simulink model "Channel_Picking_6_of_20"  (R2023a)
settings: Solver=ode23tb  StartTime=0.0  StopTime=3.0  RelTol=1e-3
libraries: dspfdesign x21, dspindex x4, dspvision x2, dspstat3 x1
settings Model: Creator=zacha  LastModifiedBy=zacha
settings DebuggingCC: UnconnectedInputMsg=warning  UnconnectedOutputMsg=warning  UnconnectedLineMsg=warning
settings ModelReferenceCC: EnableRefExpFcnMdlSchedulingChecks=on
settings RTWCC: DLArmComputeVersion=19.05

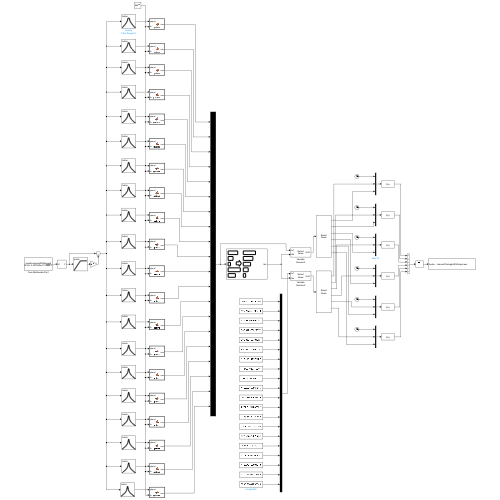
[thumbnail: Simulink's stored preview of the top-level diagram]
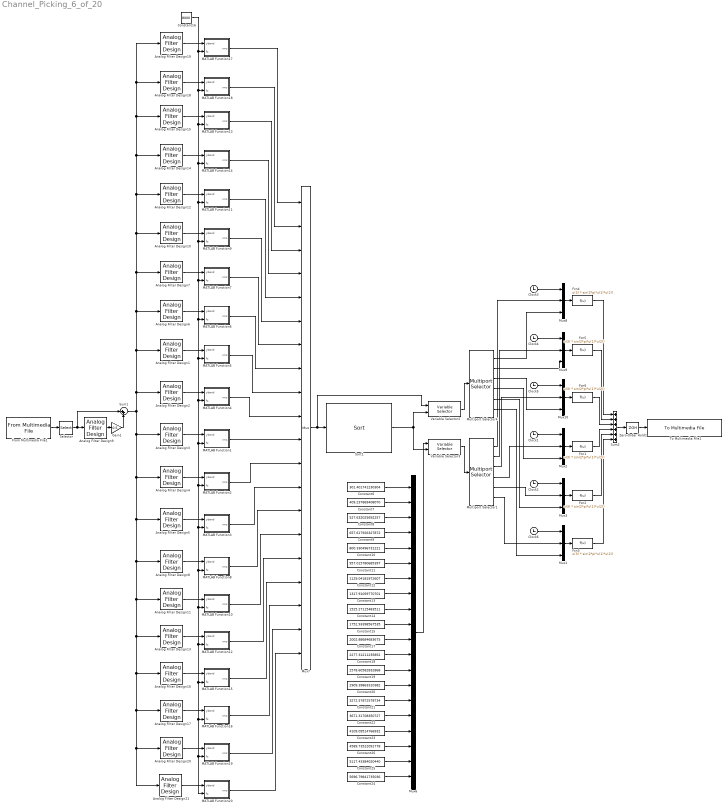
== system Channel_Picking_6_of_20 ==
  Analog Filter Design1 : dspfdesign/Analog Filter Design  method=Butterworth  filttype=Bandpass  N=6  Wlo=8901.71649069657  Whi=10265.4061283531  Rp=2  Rs=40
  Analog Filter Design10 : dspfdesign/Analog Filter Design  method=Butterworth  filttype=Bandpass  N=6  Wlo=5497.89355477605  Whi=6528.32142910693  Rp=2  Rs=40
  Analog Filter Design11 : dspfdesign/Analog Filter Design  method=Butterworth  filttype=Bandpass  N=6  Wlo=19368.0065720074  Whi=21756.4305609036  Rp=2  Rs=40
  Analog Filter Design12 : dspfdesign/Analog Filter Design  method=Butterworth  filttype=Bandpass  N=6  Wlo=4559.35608112265  Whi=5497.89355477605  Rp=2  Rs=40
  Analog Filter Design13 : dspfdesign/Analog Filter Design  method=Butterworth  filttype=Bandpass  N=6  Wlo=21756.4305609036  Whi=24378.7005532769  Rp=2  Rs=40
  Analog Filter Design14 : dspfdesign/Analog Filter Design  method=Butterworth  filttype=Bandpass  N=6  Wlo=3704.51450375974  Whi=4559.35608112265  Rp=2  Rs=40
  Analog Filter Design15 : dspfdesign/Analog Filter Design  method=Butterworth  filttype=Bandpass  N=6  Wlo=2925.90507909423  Whi=3704.51450375974  Rp=2  Rs=40
  Analog Filter Design16 : dspfdesign/Analog Filter Design  method=Butterworth  filttype=Bandpass  N=6  Wlo=24378.7005532769  Whi=27257.7119620007  Rp=2  Rs=40
  Analog Filter Design17 : dspfdesign/Analog Filter Design  method=Butterworth  filttype=Bandpass  N=6  Wlo=27257.7119620007  Whi=30418.6018458298  Rp=2  Rs=40
  Analog Filter Design18 : dspfdesign/Analog Filter Design  method=Butterworth  filttype=Bandpass  N=6  Wlo=2216.72965731829  Whi=2925.90507909423  Rp=2  Rs=40
  Analog Filter Design19 : dspfdesign/Analog Filter Design  method=Butterworth  filttype=Bandpass  N=6  Wlo=1570.79632679490  Whi=2216.72965731829  Rp=2  Rs=40
  Analog Filter Design2 : dspfdesign/Analog Filter Design  method=Butterworth  filttype=Bandpass  N=6  Wlo=10265.4061283531  Whi=11762.6119981492  Rp=2  Rs=40
  Analog Filter Design20 : dspfdesign/Analog Filter Design  method=Butterworth  filttype=Bandpass  N=6  Wlo=30418.6018458298  Whi=33888.9683846419  Rp=2  Rs=40
  Analog Filter Design21 : dspfdesign/Analog Filter Design  method=Butterworth  filttype=Bandpass  N=6  Wlo=33888.9683846419  Whi=37699.1118430775  Rp=2  Rs=40
  Analog Filter Design3 : dspfdesign/Analog Filter Design  method=Butterworth  filttype=Bandpass  N=6  Wlo=11762.6119981492  Whi=13406.4064178267  Rp=2  Rs=40
  Analog Filter Design4 : dspfdesign/Analog Filter Design  method=Butterworth  filttype=Bandpass  N=6  Wlo=13406.4064178267  Whi=15211.1415906396  Rp=2  Rs=40
  Analog Filter Design5 : dspfdesign/Analog Filter Design  method=Butterworth  filttype=Bandpass  N=6  Wlo=15211.1415906396  Whi=17192.5749164852  Rp=2  Rs=40
  Analog Filter Design6 : dspfdesign/Analog Filter Design  method=Butterworth  filttype=Bandpass  N=6  Wlo=7659.63651668133  Whi=8901.71649069657  Rp=2  Rs=40
  Analog Filter Design7 : dspfdesign/Analog Filter Design  method=Butterworth  filttype=Bandpass  N=6  Wlo=6528.32142910693  Whi=7659.63651668133  Rp=2  Rs=40
  Analog Filter Design8 : dspfdesign/Analog Filter Design  method=Butterworth  filttype=Bandpass  N=6  Wlo=17192.5749164852  Whi=19368.0065720074  Rp=2  Rs=40
  Analog Filter Design9 : dspfdesign/Analog Filter Design  method=Butterworth  filttype=Highpass  N=6  Wlo=7539.82236  Whi=80  Rp=2  Rs=40
  Clock{1..6} (6 alike) : Clock
  Constant10 : Constant  Value=800.330496731221
  Constant11 : Constant  Value=957.015780685397
  Constant12 : Constant  Value=1129.04181972607
  Constant13 : Constant  Value=1317.91059770701
  Constant14 : Constant  Value=1525.27115483511
  Constant15 : Constant  Value=1752.93398567535
  Constant16 : Constant  Value=8000
  Constant17 : Constant  Value=2002.88684683675
  Constant18 : Constant  Value=2277.31211235852
  Constant19 : Constant  Value=2578.60582832868
  Constant20 : Constant  Value=2909.39863310382
  Constant21 : Constant  Value=3272.57872578734
  Constant22 : Constant  Value=3671.31708350727
  Constant23 : Constant  Value=4109.09514766932
  Constant24 : Constant  Value=5696.79841735036
  Constant25 : Constant  Value=5117.43384020440
  Constant26 : Constant  Value=4589.73522091778
  Constant6 : Constant  Value=301.401741230304
  Constant7 : Constant  Value=409.237869408070
  Constant8 : Constant  Value=527.632025692257
  Constant9 : Constant  Value=657.617926327872
  Fcn{1..6} (6 alike) : Fcn  Expr=u(3) * sin(2*pi*u(1)*u(2))
  From Multimedia File1 : dspvision/From Multimedia File  inputFilename=C:\Users\zacha\Desktop\Cochlear\Media\inputSentance8000hz.mp3  readRange=[1 Inf]  loop=on  numPlays=1  outputStreams=Audio only  videoDataType=single  audioDataType=double  inheritSampleTime=off  userDefinedSampleTime=1/8000  noAudioOutput=off  isIntensityVideo=off  fourcc=RGB  colorVideoFormat=Separate color signals  outputEOF=off  dataOrg=Column-major  audioFrameSize=1  computeAudioFrameSize=off  outSamplingMode=Sample based
      settings: LibrarySourceBlock=dspsrcs4/From Multimedia File
  Gain1 : Gain  Gain=0.5
  MATLAB Function1 : MATLAB Function  TreatAsAtomicUnit=on
  MATLAB Function10 : MATLAB Function  TreatAsAtomicUnit=on
  MATLAB Function11 : MATLAB Function  TreatAsAtomicUnit=on
  MATLAB Function12 : MATLAB Function  TreatAsAtomicUnit=on
  MATLAB Function13 : MATLAB Function  TreatAsAtomicUnit=on
  MATLAB Function14 : MATLAB Function  TreatAsAtomicUnit=on
  MATLAB Function15 : MATLAB Function  TreatAsAtomicUnit=on
  MATLAB Function16 : MATLAB Function  TreatAsAtomicUnit=on
  MATLAB Function17 : MATLAB Function  TreatAsAtomicUnit=on
  MATLAB Function18 : MATLAB Function  TreatAsAtomicUnit=on
  MATLAB Function19 : MATLAB Function  TreatAsAtomicUnit=on
  MATLAB Function2 : MATLAB Function  TreatAsAtomicUnit=on
  MATLAB Function20 : MATLAB Function  TreatAsAtomicUnit=on
  MATLAB Function3 : MATLAB Function  TreatAsAtomicUnit=on
  MATLAB Function4 : MATLAB Function  TreatAsAtomicUnit=on
  MATLAB Function5 : MATLAB Function  TreatAsAtomicUnit=on
  MATLAB Function6 : MATLAB Function  TreatAsAtomicUnit=on
  MATLAB Function7 : MATLAB Function  TreatAsAtomicUnit=on
  MATLAB Function8 : MATLAB Function  TreatAsAtomicUnit=on
  MATLAB Function9 : MATLAB Function  TreatAsAtomicUnit=on
  Multiport Selector1 : dspindex/Multiport Selector  rowsOrCols=Rows  idxCellArray={ 1, 2,3,4,5,6 }  idxErrMode=Clip Index
  Multiport Selector4 : dspindex/Multiport Selector  rowsOrCols=Rows  idxCellArray={ 1, 2,3,4,5,6 }  idxErrMode=Clip Index
  Mux{1..3,8..10} (6 alike) : Mux  Inputs=3
  Mux6 : Mux  Inputs=20
  Mux7 : Mux  Inputs=20
  Selector : Selector  NumberOfDimensions=2  InputPortWidth=3  IndexOptions=Select all,Index vector (dialog)  Indices=[2],1  OutputSizes=1,1
  Sort1 : dspstat3/Sort  otype=Index  dir=Descending  sortAlg=Quick sort  roundingMode=Floor  overflowMode=off  accumDataTypeStr=Inherit: Same as product output  accumLastDataTypeStr=Inherit: Same as product output
  Sum1 : Sum  Inputs=|++
  Sum2 : Sum  Inputs=++++++
  To Multimedia File1 : dspvision/To Multimedia File  outputFilename=C:\Users\zacha\Desktop\Cochlear\Media\channelPicking6of20Output.wav  streamSelection=Audio only  videoCompressor=None (uncompressed)  audioCompressor=None (uncompressed)  imagePorts=Separate color signals  fileType=WAV  audioDatatype=16-bit integer  fourcc=RGB  videoQuality=75  mj2000CompFactor=10
      settings: LibrarySourceBlock=dspsnks4/To Multimedia File
  Variable Selector2 : dspindex/Variable Selector  NumInputs=1  rowsOrCols=Rows  IdxMode=Variable  Elements=[1 3]  ZerOneIdxMode=One-based  errmode=Clip Index  FillMode=on  FillValues=0
      settings: LibrarySourceBlock=|
      | dsphdlsupportsigmgmt/Variable
      | Selector
  Variable Selector3 : dspindex/Variable Selector  NumInputs=1  rowsOrCols=Rows  IdxMode=Variable  Elements=[1 3]  ZerOneIdxMode=One-based  errmode=Clip Index  FillMode=on  FillValues=0
      settings: LibrarySourceBlock=|
      | dsphdlsupportsigmgmt/Variable
      | Selector
  Zero-Order Hold1 : ZeroOrderHold  SampleTime=1/8000
  wires:
  Analog Filter Design20/1 -> MATLAB Function19/1(yband)
  Analog Filter Design21/1 -> MATLAB Function20/1(yband)
  Sum1/1 -> Analog Filter Design19/1, Analog Filter Design18/1, Analog Filter Design15/1, Analog Filter Design14/1, Analog Filter Design12/1, Analog Filter Design10/1, Analog Filter Design7/1, Analog Filter Design6/1, Analog Filter Design1/1, Analog Filter Design2/1, Analog Filter Design21/1, Analog Filter Design20/1, Analog Filter Design17/1, Analog Filter Design16/1, Analog Filter Design13/1, Analog Filter Design11/1, Analog Filter Design8/1, Analog Filter Design5/1, Analog Filter Design4/1, Analog Filter Design3/1
  Analog Filter Design8/1 -> MATLAB Function8/1(yband)
  Analog Filter Design10/1 -> MATLAB Function9/1(yband)
  Analog Filter Design6/1 -> MATLAB Function6/1(yband)
  Analog Filter Design3/1 -> MATLAB Function1/1(yband)
  Analog Filter Design13/1 -> MATLAB Function12/1(yband)
  Analog Filter Design2/1 -> MATLAB Function4/1(yband)
  Analog Filter Design15/1 -> MATLAB Function13/1(yband)
  Analog Filter Design12/1 -> MATLAB Function11/1(yband)
  Analog Filter Design4/1 -> MATLAB Function2/1(yband)
  Analog Filter Design7/1 -> MATLAB Function7/1(yband)
  Analog Filter Design11/1 -> MATLAB Function10/1(yband)
  Analog Filter Design9/1 -> Gain1/1
  Analog Filter Design19/1 -> MATLAB Function17/1(yband)
  Analog Filter Design5/1 -> MATLAB Function3/1(yband)
  Constant16/1 -> MATLAB Function20/2(fs), MATLAB Function19/2(fs), MATLAB Function16/2(fs), MATLAB Function15/2(fs), MATLAB Function12/2(fs), MATLAB Function10/2(fs), MATLAB Function8/2(fs), MATLAB Function3/2(fs), MATLAB Function2/2(fs), MATLAB Function1/2(fs), MATLAB Function4/2(fs), MATLAB Function5/2(fs), MATLAB Function6/2(fs), MATLAB Function7/2(fs), MATLAB Function9/2(fs), MATLAB Function11/2(fs), MATLAB Function14/2(fs), MATLAB Function13/2(fs), MATLAB Function18/2(fs), MATLAB Function17/2(fs)
  Analog Filter Design18/1 -> MATLAB Function18/1(yband)
  Analog Filter Design1/1 -> MATLAB Function5/1(yband)
  Analog Filter Design16/1 -> MATLAB Function15/1(yband)
  Analog Filter Design14/1 -> MATLAB Function14/1(yband)
  Analog Filter Design17/1 -> MATLAB Function16/1(yband)
  From Multimedia File1/1 -> Selector/1
  Gain1/1 -> Sum1/2
  Selector/1 -> Analog Filter Design9/1, Sum1/1
  Constant6/1 -> Mux6/1
  Constant7/1 -> Mux6/2
  Constant8/1 -> Mux6/3
  Constant9/1 -> Mux6/4
  Constant10/1 -> Mux6/5
  Constant11/1 -> Mux6/6
  Constant12/1 -> Mux6/7
  Constant13/1 -> Mux6/8
  Constant14/1 -> Mux6/9
  Constant15/1 -> Mux6/10
  Constant17/1 -> Mux6/11
  Constant18/1 -> Mux6/12
  Constant19/1 -> Mux6/13
  Constant20/1 -> Mux6/14
  Constant21/1 -> Mux6/15
  Constant22/1 -> Mux6/16
  Constant23/1 -> Mux6/17
  Constant26/1 -> Mux6/18
  Constant25/1 -> Mux6/19
  Constant24/1 -> Mux6/20
  MATLAB Function17/1(rms) -> Mux7/1
  MATLAB Function18/1(rms) -> Mux7/2
  MATLAB Function13/1(rms) -> Mux7/3
  MATLAB Function14/1(rms) -> Mux7/4
  MATLAB Function11/1(rms) -> Mux7/5
  MATLAB Function9/1(rms) -> Mux7/6
  MATLAB Function7/1(rms) -> Mux7/7
  MATLAB Function6/1(rms) -> Mux7/8
  MATLAB Function5/1(rms) -> Mux7/9
  MATLAB Function4/1(rms) -> Mux7/10
  MATLAB Function1/1(rms) -> Mux7/11
  MATLAB Function2/1(rms) -> Mux7/12
  MATLAB Function3/1(rms) -> Mux7/13
  MATLAB Function8/1(rms) -> Mux7/14
  MATLAB Function10/1(rms) -> Mux7/15
  MATLAB Function12/1(rms) -> Mux7/16
  MATLAB Function15/1(rms) -> Mux7/17
  MATLAB Function16/1(rms) -> Mux7/18
  MATLAB Function19/1(rms) -> Mux7/19
  MATLAB Function20/1(rms) -> Mux7/20
  Mux7/1 -> Variable Selector2/1, Sort1/1
  Variable Selector2/1 -> Multiport Selector4/1
  Variable Selector3/1 -> Multiport Selector1/1
  Sort1/1 -> Variable Selector2/2, Variable Selector3/2
  Mux6/1 -> Variable Selector3/1
  Mux9/1 -> Fcn5/1
  Clock4/1 -> Mux9/1
  Fcn4/1 -> Sum2/1
  Sum2/1 -> Zero-Order Hold1/1
  Clock3/1 -> Mux8/1
  Mux8/1 -> Fcn4/1
  Fcn6/1 -> Sum2/3
  Fcn5/1 -> Sum2/2
  Zero-Order Hold1/1 -> To Multimedia File1/1
  Clock5/1 -> Mux10/1
  Mux10/1 -> Fcn6/1
  Clock6/1 -> Mux1/1
  Mux3/1 -> Fcn2/1
  Mux2/1 -> Fcn1/1
  Clock2/1 -> Mux3/1
  Clock1/1 -> Mux2/1
  Mux1/1 -> Fcn3/1
  Fcn1/1 -> Sum2/4
  Fcn2/1 -> Sum2/5
  Fcn3/1 -> Sum2/6
  Multiport Selector4/1 -> Mux8/3
  Multiport Selector4/2 -> Mux9/3
  Multiport Selector4/3 -> Mux10/3
  Multiport Selector4/4 -> Mux2/3
  Multiport Selector4/5 -> Mux3/3
  Multiport Selector4/6 -> Mux1/3
  Multiport Selector1/1 -> Mux8/2
  Multiport Selector1/2 -> Mux9/2
  Multiport Selector1/3 -> Mux10/2
  Multiport Selector1/4 -> Mux2/2
  Multiport Selector1/5 -> Mux3/2
  Multiport Selector1/6 -> Mux1/2

== matlab function Channel_Picking_6_of_20/MATLAB Function13 ==
  data: yband input; rms output; fs input
function rms = getrms(yband,fs)

    y = abs(yband); %rectifying it makes it sound bad

    [b,a] = butter(2,400/(fs/2));

    z = filter(b,a,y); %this filter also makes it sound bad

    windowsize = round(4/(1000/fs)); %rms computed every 4ms = windowsize samples

    [yupper,ylower] = envelope(yband,windowsize,'rms'); %changed to yband here

    %envelope(z,windowsize,'rms');

    rms = yupper;
end

== matlab function Channel_Picking_6_of_20/MATLAB Function14 ==
  data: yband input; rms output; fs input
function rms = getrms(yband,fs)

    y = abs(yband); %rectifying it makes it sound bad

    [b,a] = butter(2,400/(fs/2));

    z = filter(b,a,y); %this filter also makes it sound bad

    windowsize = round(4/(1000/fs)); %rms computed every 4ms = windowsize samples

    [yupper,ylower] = envelope(yband,windowsize,'rms'); %changed to yband here

    %envelope(z,windowsize,'rms');

    rms = yupper;
end

== matlab function Channel_Picking_6_of_20/MATLAB Function15 ==
  data: yband input; rms output; fs input
function rms = getrms(yband,fs)

    y = abs(yband); %rectifying it makes it sound bad

    [b,a] = butter(2,400/(fs/2));

    z = filter(b,a,y); %this filter also makes it sound bad

    windowsize = round(4/(1000/fs)); %rms computed every 4ms = windowsize samples

    [yupper,ylower] = envelope(yband,windowsize,'rms'); %changed to yband here

    %envelope(z,windowsize,'rms');

    rms = yupper;
end

== matlab function Channel_Picking_6_of_20/MATLAB Function16 ==
  data: yband input; rms output; fs input
function rms = getrms(yband,fs)

    y = abs(yband); %rectifying it makes it sound bad

    [b,a] = butter(2,400/(fs/2));

    z = filter(b,a,y); %this filter also makes it sound bad

    windowsize = round(4/(1000/fs)); %rms computed every 4ms = windowsize samples

    [yupper,ylower] = envelope(yband,windowsize,'rms'); %changed to yband here

    %envelope(z,windowsize,'rms');

    rms = yupper;
end

== matlab function Channel_Picking_6_of_20/MATLAB Function17 ==
  data: yband input; rms output; fs input
function rms = getrms(yband,fs)

    y = abs(yband); %rectifying it makes it sound bad

    [b,a] = butter(2,400/(fs/2));

    z = filter(b,a,y); %this filter also makes it sound bad

    windowsize = round(4/(1000/fs)); %rms computed every 4ms = windowsize samples

    [yupper,ylower] = envelope(yband,windowsize,'rms'); %changed to yband here

    %envelope(z,windowsize,'rms');

    rms = yupper;
end

== matlab function Channel_Picking_6_of_20/MATLAB Function18 ==
  data: yband input; rms output; fs input
function rms = getrms(yband,fs)

    y = abs(yband); %rectifying it makes it sound bad

    [b,a] = butter(2,400/(fs/2));

    z = filter(b,a,y); %this filter also makes it sound bad

    windowsize = round(4/(1000/fs)); %rms computed every 4ms = windowsize samples

    [yupper,ylower] = envelope(yband,windowsize,'rms'); %changed to yband here

    %envelope(z,windowsize,'rms');

    rms = yupper;
end

== matlab function Channel_Picking_6_of_20/MATLAB Function19 ==
  data: yband input; rms output; fs input
function rms = getrms(yband,fs)

    y = abs(yband); %rectifying it makes it sound bad

    [b,a] = butter(2,400/(fs/2));

    z = filter(b,a,y); %this filter also makes it sound bad

    windowsize = round(4/(1000/fs)); %rms computed every 4ms = windowsize samples

    [yupper,ylower] = envelope(yband,windowsize,'rms'); %changed to yband here

    %envelope(z,windowsize,'rms');

    rms = yupper;
end

== matlab function Channel_Picking_6_of_20/MATLAB Function20 ==
  data: yband input; rms output; fs input
function rms = getrms(yband,fs)

    y = abs(yband); %rectifying it makes it sound bad

    [b,a] = butter(2,400/(fs/2));

    z = filter(b,a,y); %this filter also makes it sound bad

    windowsize = round(4/(1000/fs)); %rms computed every 4ms = windowsize samples

    [yupper,ylower] = envelope(yband,windowsize,'rms'); %changed to yband here

    %envelope(z,windowsize,'rms');

    rms = yupper;
end

== matlab function Channel_Picking_6_of_20/MATLAB Function2 ==
  data: yband input; rms output; fs input
function rms = getrms(yband,fs)

    y = abs(yband); %rectifying it makes it sound bad

    [b,a] = butter(2,400/(fs/2));

    z = filter(b,a,y); %this filter also makes it sound bad

    windowsize = round(4/(1000/fs)); %rms computed every 4ms = windowsize samples

    [yupper,ylower] = envelope(yband,windowsize,'rms'); %changed to yband here

    %envelope(z,windowsize,'rms');

    rms = yupper;
end

== matlab function Channel_Picking_6_of_20/MATLAB Function3 ==
  data: yband input; rms output; fs input
function rms = getrms(yband,fs)

    y = abs(yband); %rectifying it makes it sound bad

    [b,a] = butter(2,400/(fs/2));

    z = filter(b,a,y); %this filter also makes it sound bad

    windowsize = round(4/(1000/fs)); %rms computed every 4ms = windowsize samples

    [yupper,ylower] = envelope(yband,windowsize,'rms'); %changed to yband here

    %envelope(z,windowsize,'rms');

    rms = yupper;
end

== matlab function Channel_Picking_6_of_20/MATLAB Function6 ==
  data: yband input; rms output; fs input
function rms = getrms(yband,fs)

    y = abs(yband); %rectifying it makes it sound bad

    [b,a] = butter(2,400/(fs/2));

    z = filter(b,a,y); %this filter also makes it sound bad

    windowsize = round(4/(1000/fs)); %rms computed every 4ms = windowsize samples

    [yupper,ylower] = envelope(yband,windowsize,'rms'); %changed to yband here

    %envelope(z,windowsize,'rms');

    rms = yupper;
end

== matlab function Channel_Picking_6_of_20/MATLAB Function4 ==
  data: yband input; rms output; fs input
function rms = getrms(yband,fs)

    y = abs(yband); %rectifying it makes it sound bad

    [b,a] = butter(2,400/(fs/2));

    z = filter(b,a,y); %this filter also makes it sound bad

    windowsize = round(4/(1000/fs)); %rms computed every 4ms = windowsize samples

    [yupper,ylower] = envelope(yband,windowsize,'rms'); %changed to yband here

    %envelope(z,windowsize,'rms');

    rms = yupper;
end

== matlab function Channel_Picking_6_of_20/MATLAB Function5 ==
  data: yband input; rms output; fs input
function rms = getrms(yband,fs)

    y = abs(yband); %rectifying it makes it sound bad

    [b,a] = butter(2,400/(fs/2));

    z = filter(b,a,y); %this filter also makes it sound bad

    windowsize = round(4/(1000/fs)); %rms computed every 4ms = windowsize samples

    [yupper,ylower] = envelope(yband,windowsize,'rms'); %changed to yband here

    %envelope(z,windowsize,'rms');

    rms = yupper;
end

== matlab function Channel_Picking_6_of_20/MATLAB Function7 ==
  data: yband input; rms output; fs input
function rms = getrms(yband,fs)

    y = abs(yband); %rectifying it makes it sound bad

    [b,a] = butter(2,400/(fs/2));

    z = filter(b,a,y); %this filter also makes it sound bad

    windowsize = round(4/(1000/fs)); %rms computed every 4ms = windowsize samples

    [yupper,ylower] = envelope(yband,windowsize,'rms'); %changed to yband here

    %envelope(z,windowsize,'rms');

    rms = yupper;
end

== matlab function Channel_Picking_6_of_20/MATLAB Function8 ==
  data: yband input; rms output; fs input
function rms = getrms(yband,fs)

    y = abs(yband); %rectifying it makes it sound bad

    [b,a] = butter(2,400/(fs/2));

    z = filter(b,a,y); %this filter also makes it sound bad

    windowsize = round(4/(1000/fs)); %rms computed every 4ms = windowsize samples

    [yupper,ylower] = envelope(yband,windowsize,'rms'); %changed to yband here

    %envelope(z,windowsize,'rms');

    rms = yupper;
end

== matlab function Channel_Picking_6_of_20/MATLAB Function9 ==
  data: yband input; rms output; fs input
function rms = getrms(yband,fs)

    y = abs(yband); %rectifying it makes it sound bad

    [b,a] = butter(2,400/(fs/2));

    z = filter(b,a,y); %this filter also makes it sound bad

    windowsize = round(4/(1000/fs)); %rms computed every 4ms = windowsize samples

    [yupper,ylower] = envelope(yband,windowsize,'rms'); %changed to yband here

    %envelope(z,windowsize,'rms');

    rms = yupper;
end

== matlab function Channel_Picking_6_of_20/MATLAB Function10 ==
  data: yband input; rms output; fs input
function rms = getrms(yband,fs)

    y = abs(yband); %rectifying it makes it sound bad

    [b,a] = butter(2,400/(fs/2));

    z = filter(b,a,y); %this filter also makes it sound bad

    windowsize = round(4/(1000/fs)); %rms computed every 4ms = windowsize samples

    [yupper,ylower] = envelope(yband,windowsize,'rms'); %changed to yband here

    %envelope(z,windowsize,'rms');

    rms = yupper;
end

== matlab function Channel_Picking_6_of_20/MATLAB Function11 ==
  data: yband input; rms output; fs input
function rms = getrms(yband,fs)

    y = abs(yband); %rectifying it makes it sound bad

    [b,a] = butter(2,400/(fs/2));

    z = filter(b,a,y); %this filter also makes it sound bad

    windowsize = round(4/(1000/fs)); %rms computed every 4ms = windowsize samples

    [yupper,ylower] = envelope(yband,windowsize,'rms'); %changed to yband here

    %envelope(z,windowsize,'rms');

    rms = yupper;
end

== matlab function Channel_Picking_6_of_20/MATLAB Function1 ==
  data: yband input; rms output; fs input
function rms = getrms(yband,fs)

    y = abs(yband); %rectifying it makes it sound bad

    [b,a] = butter(2,400/(fs/2));

    z = filter(b,a,y); %this filter also makes it sound bad

    windowsize = round(4/(1000/fs)); %rms computed every 4ms = windowsize samples

    [yupper,ylower] = envelope(yband,windowsize,'rms'); %changed to yband here

    %envelope(z,windowsize,'rms');

    rms = yupper;
end

== matlab function Channel_Picking_6_of_20/MATLAB Function12 ==
  data: yband input; rms output; fs input
function rms = getrms(yband,fs)

    y = abs(yband); %rectifying it makes it sound bad

    [b,a] = butter(2,400/(fs/2));

    z = filter(b,a,y); %this filter also makes it sound bad

    windowsize = round(4/(1000/fs)); %rms computed every 4ms = windowsize samples

    [yupper,ylower] = envelope(yband,windowsize,'rms'); %changed to yband here

    %envelope(z,windowsize,'rms');

    rms = yupper;
end
